simulink model "rtwdemo_fcnprotoctrl"  (Simulink 7.6)
settings: Solver=FixedStepDiscrete  StartTime=0.0  StopTime=10.0  RelTol=1e-3  SampleTimeConstraint=STIndependent
PostLoadFcn:
  | rtwdemo_fcnprotoctrl_data
libraries: rtwdemowidgets x2
Description:
  | Specifying Function Prototypes for Models
CloseFcn:
  | rtwprivate ssgencode ModelCloseRequest usability_fcnprotoctl
settings Model: Creator=The MathWorks Inc.  CovMetricSettings=d  ExtModeAutoUpdateStatusClock=off
settings DataIOCC: SaveOutput=off  SaveTime=off  SignalLoggingName=sigsOut
settings OptimizationCC: InlineParams=on  InlineInvariantSignals=on  PassReuseOutputArgsAs=Individual arguments  StateBitsets=on  DataBitsets=on  UseTempVars=on  ZeroExternalMemoryAtStartup=off  ZeroInternalMemoryAtStartup=off  NoFixptDivByZeroProtection=on  EfficientFloat2IntCast=on  EfficientMapNaN2IntZero=off  OptimizeModelRefInitCode=on  LifeSpan=1
settings DebuggingCC: CheckExecutionContextPreStartOutputMsg=on  CheckExecutionContextRuntimeOutputMsg=on  SolverPrmCheckMsg=none  ParameterUnderflowMsg=error  ParameterPrecisionLossMsg=none  StrictBusMsg=ErrorOnBusTreatedAsVector
settings HardwareCC: ProdBitPerLong=64  ProdEndianess=LittleEndian  ProdWordSize=64  ProdHWDeviceType=Specified  TargetHWDeviceType=Generic->32-bit Embedded Processor
settings SFSimCC: SimParseCustomCode=off
settings RTWCC: SystemTargetFile=ert.tlc  TLCOptions=-p0  TemplateMakefile=ert_default_tmf  Description=Real-Time Workshop Embedded Coder (no auto configuration)  GenerateReport=on  RTWVerbose=off  ProcessScript=ert_make_rtw_hook  IncludeHyperlinkInReport=on  LaunchReport=on  GenerateTraceInfo=on  GenerateTraceReport=on  GenerateTraceReportSl=on  GenerateTraceReportSf=on  GenerateTraceReportEml=on
settings CodeAppCC: ForceParamTrailComments=on  IgnoreCustomStorageClasses=off  IgnoreTestpoints=on  SimulinkDataObjDesc=on  CustomSymbolStrGlobalVar=rt$N$M  CustomSymbolStrType=$N$M  CustomSymbolStrFcn=$N$M$F  CustomSymbolStrMacro=$N$M  InsertBlockDesc=on
settings ERTTargetCC: MultiwordLength=2048  GenerateSampleERTMain=on  IncludeMdlTerminateFcn=off  SupportNonFinite=off  SupportComplex=off  InlinedParameterPlacement=NonHierarchical  ERTCustomFileTemplate=example_file_process.tlc  ConvertIfToSwitch=off

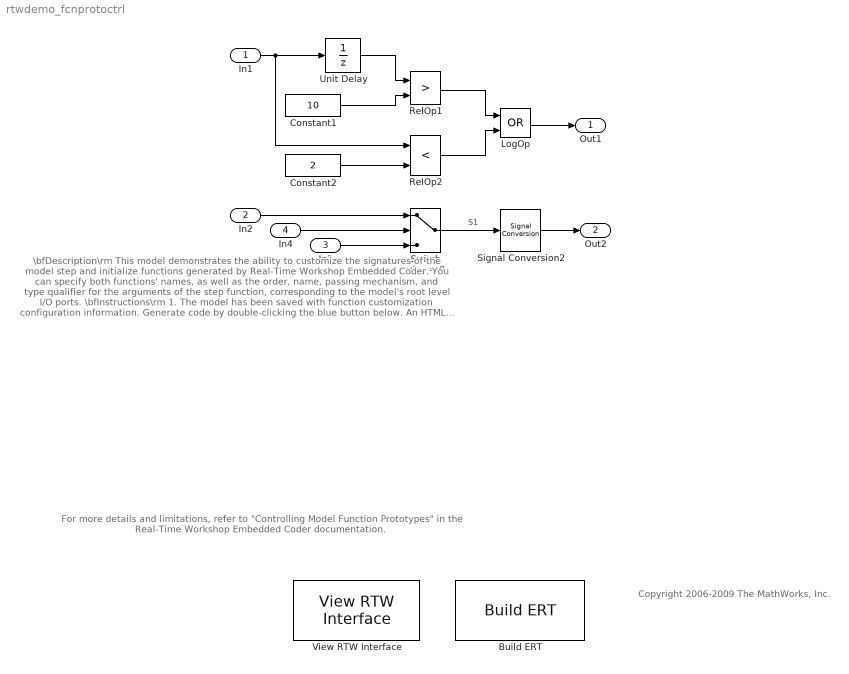
== system rtwdemo_fcnprotoctrl ==
  note: \bfDescription\rm
      | This model demonstrates the ability to customize the signatures of the model step and initialize functions
      | generated by Real-Time Workshop Embedded Coder. You can specify both functions' names, as well as
      | the order, name, passing mechanism, and type qualifier for the arguments of the step function,
      | corresponding to the model's root level I/O ports.
      |
      | \bfInstructions\rm
      | 1. The model has been saved with function customization configuration information. Generate
      |     code by double-clicking the blue button below.  An HTML report is displayed automatically.
      | 2. Inspect the source in the generated files using the hyperlinks embedded in the report, including the
      |     customized model step and initialization functions "rtwdemo\_fcnprotoctrl\_step\_custom" and
      |     "rtwdemo\_fcnprotoctrl\_init\_custom" inside the file rtwdemo\_fcnprotoctrl.c.
      | 3. To view or change the customization configuration, double-click the yellow button below, and on the
      |     Interface pane, click "Configure Model Functions".
  note: Copyright 2006-2009 The MathWorks, Inc.
  note: For more details and limitations, refer to "Controlling Model Function Prototypes"  in the
      | Real-Time Workshop Embedded Coder documentation.
  In1 : Inport  OutDataTypeStr=double  PortDimensions=1
  In2 : Inport  Port=2  OutDataTypeStr=Bus: BusObject  BusOutputAsStruct=on
  In3 : Inport  Port=3  OutDataTypeStr=Bus: BusObject  BusOutputAsStruct=on
  In4 : Inport  Port=4  OutDataTypeStr=uint8  PortDimensions=1
  Build ERT : rtwdemowidgets/Build ERT  SystemSampleTime=-1  attrib_overrides={}
  Constant1 : Constant  Value=10  OutDataTypeStr=Inherit: Inherit via back propagation
  Constant2 : Constant  Value=2  OutDataTypeStr=Inherit: Inherit via back propagation
  LogOp : Logic  Operator=OR
  RelOp1 : RelationalOperator  Operator=>  InputSameDT=on
  RelOp2 : RelationalOperator  Operator=<  InputSameDT=on
  Signal Conversion2 : SignalConversion  ConversionOutput=Virtual bus
  Switch : Switch  Criteria=u2 ~= 0  ZeroCross=off
  Unit Delay : UnitDelay  X0=10  SampleTime=-1
  View RTW Interface : rtwdemowidgets/View RTW Interface  SystemSampleTime=-1
  Out1 : Outport
  Out2 : Outport  Port=2  OutDataTypeStr=Bus: BusObject
  wires:
  RelOp1/1 -> LogOp/1
  RelOp2/1 -> LogOp/2
  Constant2/1 -> RelOp2/2
  Constant1/1 -> RelOp1/2
  In1/1 -> RelOp2/1, Unit Delay/1
  LogOp/1 -> Out1/1
  In2/1 -> Switch/1
  Switch/1 -> Signal Conversion2/1  "S1"
  Signal Conversion2/1 -> Out2/1
  In3/1 -> Switch/3
  In4/1 -> Switch/2
  Unit Delay/1 -> RelOp1/1
